simulink library "bus_stubs_template"  (R2016b)
settings: Solver=VariableStepAuto  StartTime=0.0  StopTime=10.0  RelTol=1e-3  EnableMultiTasking=on
settings Model: Creator=Jake  LastModifiedBy=Taylor
settings DataIOCC: LimitDataPoints=on
settings OptimizationCC: LifeSpan=inf
settings DebuggingCC: AllowSymbolicDim=off  SFUnexpectedBacktrackingDiag=warning  SFNoUnconditionalDefaultTransitionDiag=warning  SFExecutionAtInitializationDiag=none
settings ModelReferenceCC: PropagateSignalLabelsOutOfModel=off
settings GRTTargetCC: TargetLangStandard=C89/C90 (ANSI)
settings ConfigComp: CovMetricSettings=dw  CovHtmlReporting=on  CovSaveCumulativeToWorkspaceVar=on  CovSaveSingleToWorkspaceVar=on  CovExternalEMLEnable=off

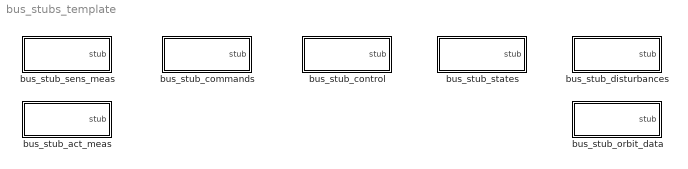
== system bus_stubs_template ==
  bus_stub_act_meas : Subsystem  mask(bus_stub_measurements){}
      mask help: Creates bus compliant with the measurements bus object.
      mask Help: Provides a zeroed bus which complies with the measurement bus object.
      mask DialogControl DescGroupVar Prompt: bus_stub_measurements
      mask DialogControl DescTextVar Prompt: Creates bus compliant with the measurements bus object.
  bus_stub_commands : Subsystem
      mask help: Creates bus compliant with actuatorCmd (actuator command) bus object.
      mask Help: Provides a zeroed bus which complies with the actuatorCmd bus object.
      mask DialogControl DescGroupVar Prompt: bus_stub_actCmd
      mask DialogControl DescTextVar Prompt: Creates bus compliant with actuatorCmd (actuator command) bus object.
  bus_stub_control : Subsystem  mask(bus_stub_actState){}
      mask help: Provides a zeroed bus which complies with the actuatorState bus object.
      mask Help: Provides a zeroed bus which complies with the actuatorState bus object.
      mask DialogControl DescGroupVar Prompt: bus_stub_actState
      mask DialogControl DescTextVar Prompt: Provides a zeroed bus which complies with the actuatorState bus object.
  bus_stub_disturbances : Subsystem  mask(bus_stub_env){}
      mask help: Creates bus compliant with the environment bus object.
      mask Help: Provides a zeroed bus which complies with the environment bus object.
      mask DialogControl DescGroupVar Prompt: bus_stub_env
      mask DialogControl DescTextVar Prompt: Creates bus compliant with the environment bus object.
  bus_stub_orbit_data : Subsystem  mask(bus_stub_env){}
      mask help: Creates bus compliant with the environment bus object.
      mask Help: Provides a zeroed bus which complies with the environment bus object.
      mask DialogControl DescGroupVar Prompt: bus_stub_env
      mask DialogControl DescTextVar Prompt: Creates bus compliant with the environment bus object.
  bus_stub_sens_meas : Subsystem  mask(bus_stub_measurements){}
      mask help: Creates bus compliant with the measurements bus object.
      mask Help: Provides a zeroed bus which complies with the measurement bus object.
      mask DialogControl DescGroupVar Prompt: bus_stub_measurements
      mask DialogControl DescTextVar Prompt: Creates bus compliant with the measurements bus object.
  bus_stub_states : Subsystem  mask(bus_stub_state){}
      mask help: Creates bus compliant with the state bus object.
      mask Help: Provides a zeroed bus which complies with the state bus object.
      mask DialogControl DescGroupVar Prompt: bus_stub_state
      mask DialogControl DescTextVar Prompt: Creates bus compliant with the state bus object.

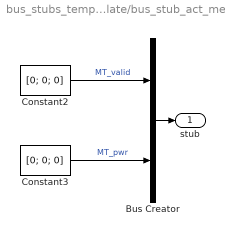
== system bus_stubs_template/bus_stub_act_meas ==
  Bus Creator : BusCreator  Inputs=2
  Constant2 : Constant  Value=[0; 0; 0]  OutDataTypeStr=boolean
  Constant3 : Constant  Value=[0; 0; 0]  OutDataTypeStr=boolean
  stub : Outport  OutDataTypeStr=Bus: act_meas
  wires:
  Bus Creator/1 -> stub/1
  Constant3/1 -> Bus Creator/2  "MT_pwr"
  Constant2/1 -> Bus Creator/1  "MT_valid"

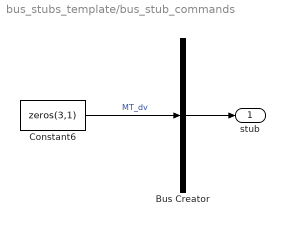
== system bus_stubs_template/bus_stub_commands ==
  Bus Creator : BusCreator  Inputs=1
  Constant6 : Constant  Value=zeros(3,1)  OutDataTypeStr=int8
  stub : Outport  OutDataTypeStr=Bus: commands
  wires:
  Bus Creator/1 -> stub/1
  Constant6/1 -> Bus Creator/1  "MT_dv"

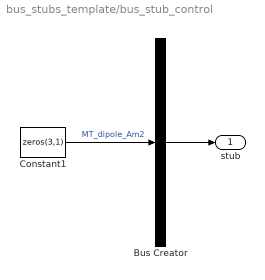
== system bus_stubs_template/bus_stub_control ==
  Bus Creator : BusCreator  Inputs=1
  Constant1 : Constant  Value=zeros(3,1)
  stub : Outport  OutDataTypeStr=Bus: control
  wires:
  Bus Creator/1 -> stub/1
  Constant1/1 -> Bus Creator/1  "MT_dipole_Am2"

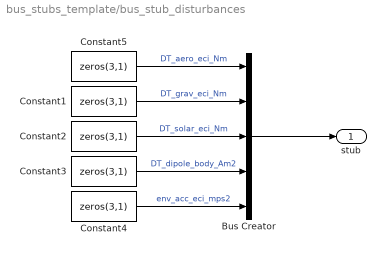
== system bus_stubs_template/bus_stub_disturbances ==
  Bus Creator : BusCreator  Inputs=5
  Constant{1..5} (5 alike) : Constant  Value=zeros(3,1)
  stub : Outport  OutDataTypeStr=Bus: disturbances
  wires:
  Bus Creator/1 -> stub/1
  Constant5/1 -> Bus Creator/1  "DT_aero_eci_Nm"
  Constant1/1 -> Bus Creator/2  "DT_grav_eci_Nm"
  Constant2/1 -> Bus Creator/3  "DT_solar_eci_Nm"
  Constant3/1 -> Bus Creator/4  "DT_dipole_body_Am2"
  Constant4/1 -> Bus Creator/5  "env_acc_eci_mps2"

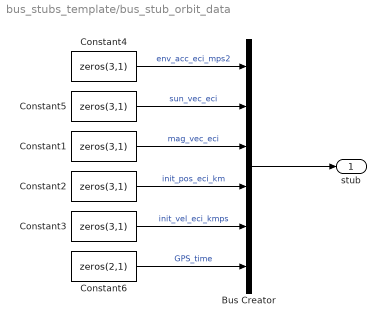
== system bus_stubs_template/bus_stub_orbit_data ==
  Bus Creator : BusCreator  Inputs=6
  Constant{1..5} (5 alike) : Constant  Value=zeros(3,1)
  Constant6 : Constant  Value=zeros(2,1)
  stub : Outport  OutDataTypeStr=Bus: orbit_data
  wires:
  Constant3/1 -> Bus Creator/5  "init_vel_eci_kmps"
  Constant2/1 -> Bus Creator/4  "init_pos_eci_km"
  Constant1/1 -> Bus Creator/3  "mag_vec_eci"
  Constant5/1 -> Bus Creator/2  "sun_vec_eci"
  Bus Creator/1 -> stub/1
  Constant4/1 -> Bus Creator/1  "env_acc_eci_mps2"
  Constant6/1 -> Bus Creator/6  "GPS_time"

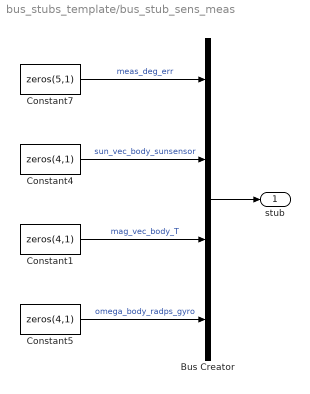
== system bus_stubs_template/bus_stub_sens_meas ==
  Bus Creator : BusCreator  Inputs=4
  Constant1 : Constant  Value=zeros(4,1)
  Constant4 : Constant  Value=zeros(4,1)
  Constant5 : Constant  Value=zeros(4,1)
  Constant7 : Constant  Value=zeros(5,1)
  stub : Outport  OutDataTypeStr=Bus: sens_meas
  wires:
  Constant4/1 -> Bus Creator/2  "sun_vec_body_sunsensor"
  Bus Creator/1 -> stub/1
  Constant1/1 -> Bus Creator/3  "mag_vec_body_T"
  Constant5/1 -> Bus Creator/4  "omega_body_radps_gyro"
  Constant7/1 -> Bus Creator/1  "meas_deg_err"

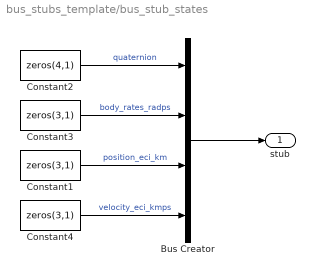
== system bus_stubs_template/bus_stub_states ==
  Bus Creator : BusCreator  Inputs=4
  Constant1 : Constant  Value=zeros(3,1)
  Constant2 : Constant  Value=zeros(4,1)
  Constant3 : Constant  Value=zeros(3,1)
  Constant4 : Constant  Value=zeros(3,1)
  stub : Outport  OutDataTypeStr=Bus: states
  wires:
  Bus Creator/1 -> stub/1
  Constant2/1 -> Bus Creator/1  "quaternion"
  Constant3/1 -> Bus Creator/2  "body_rates_radps"
  Constant1/1 -> Bus Creator/3  "position_eci_km"
  Constant4/1 -> Bus Creator/4  "velocity_eci_kmps"
